simulink model "Lab06Exp"  (Simulink 7.1)
settings: Solver=ode45  StartTime=0.0  StopTime=10.0  RelTol=1e-3
libraries: simulink x12
settings Model: Creator=George  LastModifiedBy=George

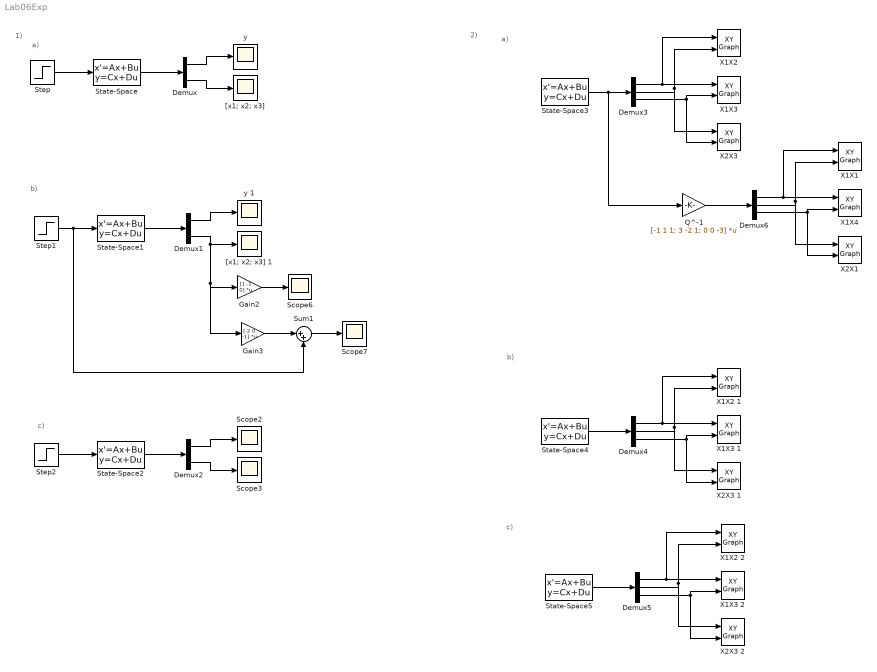
== system Lab06Exp ==
  note: a)
  note: b)
  note: c)
  note: 1)
  note: 2)
  note: a)
  note: b)
  note: c)
  Demux : Demux  Outputs=[1 3]
  Demux1 : Demux  Outputs=[1 3]
  Demux2 : Demux  Outputs=[1 3]
  Demux{3..6} (4 alike) : Demux  Outputs=3
  Gain2 : Gain  Gain=[1 -1 0]  Multiplication=Matrix(K*u) (u vector)  ParameterDataType=sfix(16)  ParameterScaling=2^0  OutDataType=sfix(16)  OutScaling=2^0
  Gain3 : Gain  Gain=[-2 0 -1]  Multiplication=Matrix(K*u) (u vector)  ParameterDataType=sfix(16)  ParameterScaling=2^0  OutDataType=sfix(16)  OutScaling=2^0
  Q^-1 : Gain  Gain=[-1 1 1; 3 -2 1; 0 0 -3]  Multiplication=Matrix(K*u) (u vector)  ParameterDataType=sfix(16)  ParameterScaling=2^0  OutDataType=sfix(16)  OutScaling=2^0
  Scope{2..3,6..7} (4 alike) : Scope
      Scope2 settings: SaveName=ScopeData2
      Scope3 settings: SaveName=ScopeData3
      Scope6 settings: SaveName=ScopeData6
      Scope7 settings: SaveName=ScopeData7
  State-Space : StateSpace  A=[-4 0 -2; 0 -4 1; 8/3 -8/3 0]  B=[2; 0; 0]  C=[0 4 0; 1 0 0; 0 1 0; 0 0 1]  D=[0; 0; 0; 0]
  State-Space1 : StateSpace  A=[-4 0 -2; 0 -4 1; 8/3 -8/3 0]  B=[2; 0; 0]  C=[0 4 0; 1 0 0; 0 1 0; 0 0 1]  D=[0; 0; 0; 0]
  State-Space2 : StateSpace  A=[0 4 0; 0 -16 4; 32/3 160/3 -16]*[-4 0 -2; 0 -4 1; 8/3 -8/3 0]*inv([0 4 0; 0 -16 4; 32/3 160/3 -16])  B=[0 4 0; 0 -16 4; 32/3 160/3 -16]*[2; 0; 0]  C=[1 0 0; 1 0 0; 0 1 0; 0 0 1]  D=[0; 0; 0; 0]
  State-Space3 : StateSpace  A=[-4 2 -1; -3 1 0; 0 0 -2]  B=[0; 0; 0]  C=[1 0 0; 0 1 0; 0 0 1]  D=[0; 0; 0]  X0=[4; -5; 1]
  State-Space4 : StateSpace  A=[-4 2 -1; -3 1 0; 0 0 -2]  B=[0; 0; 0]  C=[1 0 0; 0 1 0; 0 0 1]  D=[0; 0; 0]  X0=[4; 6; 0]
  State-Space5 : StateSpace  A=[-4 2 -1; -3 1 0; 0 0 -2]  B=[0; 0; 0]  C=[1 0 0; 0 1 0; 0 0 1]  D=[3; 4; -1]
  Step : Step  SampleTime=0
  Step1 : Step  SampleTime=0
  Step2 : Step  SampleTime=0
  Sum1 : Sum  Inputs=|++  OutDataType=sfix(16)  OutScaling=2^0
  X1X{1..4} (4 alike) : simulink/Sinks/XY Graph  SystemSampleTime=-1  xmin=-1  xmax=1  ymin=-1  ymax=1  st=-1
  X1X2 1 : simulink/Sinks/XY Graph  SystemSampleTime=-1  xmin=-1  xmax=1  ymin=-1  ymax=1  st=-1
  X1X2 2 : simulink/Sinks/XY Graph  SystemSampleTime=-1  xmin=-1  xmax=1  ymin=-1  ymax=1  st=-1
  X1X3 1 : simulink/Sinks/XY Graph  SystemSampleTime=-1  xmin=-1  xmax=1  ymin=-1  ymax=1  st=-1
  X1X3 2 : simulink/Sinks/XY Graph  SystemSampleTime=-1  xmin=-1  xmax=1  ymin=-1  ymax=1  st=-1
  X2X1 : simulink/Sinks/XY Graph  SystemSampleTime=-1  xmin=-1  xmax=1  ymin=-1  ymax=1  st=-1
  X2X3 : simulink/Sinks/XY Graph  SystemSampleTime=-1  xmin=-1  xmax=1  ymin=-1  ymax=1  st=-1
  X2X3 1 : simulink/Sinks/XY Graph  SystemSampleTime=-1  xmin=-1  xmax=1  ymin=-1  ymax=1  st=-1
  X2X3 2 : simulink/Sinks/XY Graph  SystemSampleTime=-1  xmin=-1  xmax=1  ymin=-1  ymax=1  st=-1
  "[x1; x2; x3]" : Scope
  "[x1; x2; x3] 1" : Scope
      settings: SaveName=ScopeData5
  y : Scope
  y 1 : Scope
      settings: SaveName=ScopeData4
  wires:
  Step/1 -> State-Space/1
  State-Space/1 -> Demux/1
  Demux/1 -> y/1
  Demux/2 -> "[x1; x2; x3]"/1
  Step1/1 -> State-Space1/1, Sum1/2
  State-Space1/1 -> Demux1/1
  Demux1/1 -> y 1/1
  Demux1/2 -> "[x1; x2; x3] 1"/1, Gain2/1, Gain3/1
  Gain2/1 -> Scope6/1
  Gain3/1 -> Sum1/1
  Sum1/1 -> Scope7/1
  Step2/1 -> State-Space2/1
  State-Space2/1 -> Demux2/1
  Demux2/1 -> Scope2/1
  Demux2/2 -> Scope3/1
  State-Space3/1 -> Demux3/1, Q^-1/1
  Demux3/1 -> X1X2/1, X1X3/1
  Demux3/2 -> X1X2/2, X2X3/1
  Demux3/3 -> X1X3/2, X2X3/2
  State-Space4/1 -> Demux4/1
  Demux4/1 -> X1X2 1/1, X1X3 1/1
  Demux4/2 -> X1X2 1/2, X2X3 1/1
  Demux4/3 -> X1X3 1/2, X2X3 1/2
  State-Space5/1 -> Demux5/1
  Demux5/1 -> X1X2 2/1, X1X3 2/1
  Demux5/2 -> X1X2 2/2, X2X3 2/1
  Demux5/3 -> X1X3 2/2, X2X3 2/2
  Demux6/1 -> X1X1/1, X1X4/1
  Demux6/2 -> X1X1/2, X2X1/1
  Demux6/3 -> X1X4/2, X2X1/2
  Q^-1/1 -> Demux6/1
